simulink model "BSC_sfun"  (R2015b)
settings: Solver=FixedStepDiscrete  StartTime=0.0  StopTime=inf  FixedStep=bsck_stepSize  RelTol=1e-3
settings Model: TunableVars=bscv_LowFaultType,bscv_MediumFaultType,bscv_SevereFaultType  TunableVarsStorageClass=Auto,Auto,Auto  TunableVarsTypeQualifier=,,  Creator=nctzv8  LastModifiedBy=nctzv8
settings ConfigSet: Description=OpenECU configuration set for code generation under RTW-EC.
settings SolverCC: PositivePriorityOrder=on
settings DataIOCC: SaveFormat=Array  SignalLoggingSaveFormat=ModelDataLogs
settings OptimizationCC: DefaultParameterBehavior=Inlined  InlineInvariantSignals=on  ExpressionDepthLimit=2147483647  StateBitsets=on  DataBitsets=on  ZeroExternalMemoryAtStartup=off  ZeroInternalMemoryAtStartup=off  NoFixptDivByZeroProtection=on  EfficientFloat2IntCast=on  OptimizeModelRefInitCode=on  LifeSpan=1
settings DebuggingCC: SaveWithParameterizedLinksMsg=none  UnderspecifiedInitializationDetection=Classic  MergeDetectMultiDrivingBlocksExec=none  SignalResolutionControl=TryResolveAllWithWarning  MultiTaskDSMMsg=warning  MultiTaskCondExecSysMsg=none  SingleTaskRateTransMsg=error  CheckMatrixSingularityMsg=warning  VectorMatrixConversionMsg=warning  FcnCallInpInsideContextMsg=UseLocalSettings  SignalLabelMismatchMsg=warning  StateNameClashWarn=warning  StrictBusMsg=None
settings HardwareCC: ProdBitPerPointer=32  ProdLargestAtomicInteger=Long  ProdLargestAtomicFloat=Double  ProdEndianess=BigEndian  ProdWordSize=32  ProdHWDeviceType=Freescale->32-bit PowerPC  TargetIntDivRoundTo=Zero  TargetEndianess=BigEndian  TargetHWDeviceType=Freescale->32-bit PowerPC  ProdEqTarget=off
settings RTWCC: SystemTargetFile=openecu_ert.tlc  MakeCommand=make_rtw optimized_floating_point=1  TemplateMakefile=openecu_ert_r2015b_64.tmf  Description=OpenECU Platform Target (ERT, optimised floating-point code)  RetainRTWFile=on  IncludeHyperlinkInReport=on
settings CodeAppCC: ForceParamTrailComments=on  IgnoreCustomStorageClasses=off  SimulinkDataObjDesc=on  CustomSymbolStrType=$N$R$M  InsertBlockDesc=on  InternalIdentifier=Classic
settings STFCustomTargetCC: TargetLibSuffix=.a  GenerateSampleERTMain=on  ConcurrentExecutionCompliant=off  IncludeMdlTerminateFcn=off  GeneratePreprocessorConditionals=Use local settings  CombineOutputUpdateFcns=on  IncludeFileDelimiter=UseQuote  ERTCustomFileBanners=on  SupportContinuousTime=off  MATLABClassNameForMDSCustomization=Simulink.SoftwareTarget.ERTCustomization  CPPClassGenCompliant=off  GRTInterface=off  SystemTargetFile=openecu_ert.tlc
settings ERTTargetCC: GenerateSampleERTMain=on  ParMdlRefBuildCompliant=off  CompOptLevelCompliant=off  ConcurrentExecutionCompliant=off  IncludeMdlTerminateFcn=off  ERTFirstTimeCompliant=off  IncludeFileDelimiter=UseQuote  SupportNonInlinedSFcns=on  ModelStepFunctionPrototypeControlCompliant=off  CPPClassGenCompliant=off  UseToolchainInfoCompliant=off  ExtModeMexFile=noextcomm  InlinedParameterPlacement=NonHierarchical  ERTSrcFileBannerTemplate=oe_code_c_template.cgt  ERTHdrFileBannerTemplate=oe_code_h_template.cgt  ERTDataSrcFileTemplate=oe_data_c_template.cgt  ERTDataHdrFileTemplate=oe_data_h_template.cgt  ERTCustomFileTemplate=example_file_process.tlc  GlobalDataDefinition=InSeparateSourceFile  GlobalDataReference=InSeparateHeaderFile  EnableUserReplacementTypes=on

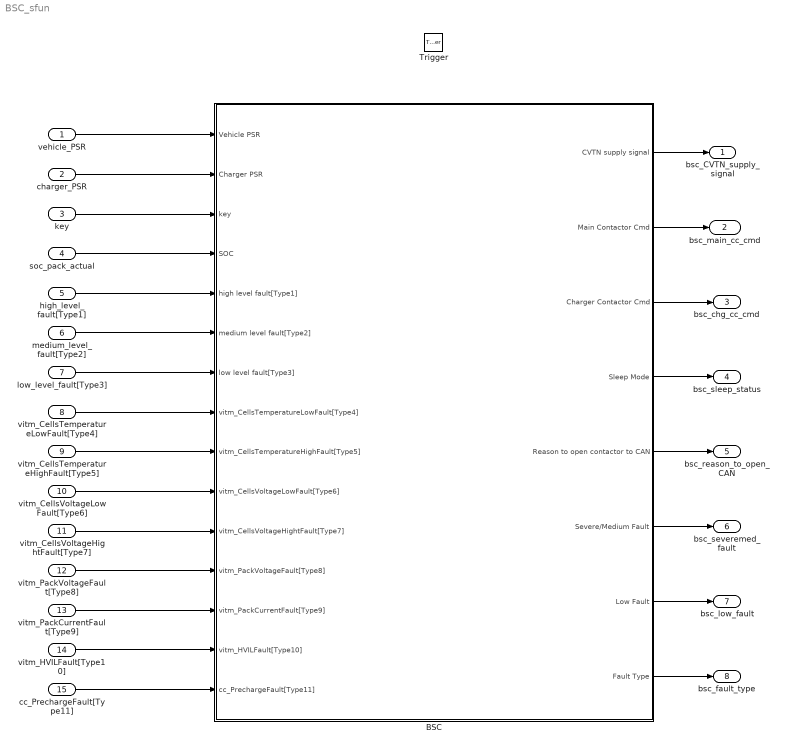
== system BSC_sfun ==
  vehicle_PSR : Inport  OutDataTypeStr=uint8  PortDimensions=1
  charger_PSR : Inport  Port=2  OutDataTypeStr=uint8  PortDimensions=1
  key : Inport  Port=3  OutDataTypeStr=uint8  PortDimensions=1
  soc_pack_actual : Inport  Port=4  OutDataTypeStr=double  PortDimensions=1
  high_level_fault[Type1] : Inport  Port=5  OutDataTypeStr=uint8  PortDimensions=1
  medium_level_fault[Type2] : Inport  Port=6  OutDataTypeStr=uint8  PortDimensions=1
  low_level_fault[Type3] : Inport  Port=7  OutDataTypeStr=uint8  PortDimensions=1
  vitm_CellsTemperatureLowFault[Type4] : Inport  Port=8  OutDataTypeStr=uint8  PortDimensions=1
  vitm_CellsTemperatureHighFault[Type5] : Inport  Port=9  OutDataTypeStr=uint8  PortDimensions=1
  vitm_CellsVoltageLowFault[Type6] : Inport  Port=10  OutDataTypeStr=uint8  PortDimensions=1
  vitm_CellsVoltageHightFault[Type7] : Inport  Port=11  OutDataTypeStr=uint8  PortDimensions=1
  vitm_PackVoltageFault[Type8] : Inport  Port=12  OutDataTypeStr=uint8  PortDimensions=1
  vitm_PackCurrentFault[Type9] : Inport  Port=13  OutDataTypeStr=uint8  PortDimensions=1
  vitm_HVILFault[Type10] : Inport  Port=14  OutDataTypeStr=uint8  PortDimensions=1
  cc_PrechargeFault[Type11] : Inport  Port=15  OutDataTypeStr=uint8  PortDimensions=1
  Trigger : TriggerPort  TriggerType=function-call  PortDimensions=1
  BSC : Subsystem
      mask help: Simulink:masks:GenSFuncDesc_MD
      mask Help: eval('feval(''rtwprivate'',''rtwhelpview'',''rtw_sfcn_block'')');
  bsc_CVTN_supply_signal : Outport  OutDataTypeStr=boolean  PortDimensions=1
  bsc_main_cc_cmd : Outport  Port=2  OutDataTypeStr=boolean  PortDimensions=1
  bsc_chg_cc_cmd : Outport  Port=3  OutDataTypeStr=boolean  PortDimensions=1
  bsc_sleep_status : Outport  Port=4  OutDataTypeStr=boolean  PortDimensions=1
  bsc_reason_to_open_CAN : Outport  Port=5  OutDataTypeStr=uint8  PortDimensions=1
  bsc_severemed_fault : Outport  Port=6  OutDataTypeStr=uint8  PortDimensions=1
  bsc_low_fault : Outport  Port=7  OutDataTypeStr=uint8  PortDimensions=1
  bsc_fault_type : Outport  Port=8  OutDataTypeStr=uint8  PortDimensions=1
  wires:
  vehicle_PSR/1 -> BSC/1(Vehicle PSR)
  charger_PSR/1 -> BSC/2(Charger PSR)
  key/1 -> BSC/3(key)
  soc_pack_actual/1 -> BSC/4(SOC)
  high_level_fault[Type1]/1 -> BSC/5(high level fault[Type1])
  medium_level_fault[Type2]/1 -> BSC/6(medium level fault[Type2])
  low_level_fault[Type3]/1 -> BSC/7(low level fault[Type3])
  vitm_CellsTemperatureLowFault[Type4]/1 -> BSC/8(vitm_CellsTemperatureLowFault[Type4])
  vitm_CellsTemperatureHighFault[Type5]/1 -> BSC/9(vitm_CellsTemperatureHighFault[Type5])
  vitm_CellsVoltageLowFault[Type6]/1 -> BSC/10(vitm_CellsVoltageLowFault[Type6])
  vitm_CellsVoltageHightFault[Type7]/1 -> BSC/11(vitm_CellsVoltageHightFault[Type7])
  vitm_PackVoltageFault[Type8]/1 -> BSC/12(vitm_PackVoltageFault[Type8])
  vitm_PackCurrentFault[Type9]/1 -> BSC/13(vitm_PackCurrentFault[Type9])
  cc_PrechargeFault[Type11]/1 -> BSC/15(cc_PrechargeFault[Type11])
  vitm_HVILFault[Type10]/1 -> BSC/14(vitm_HVILFault[Type10])
  BSC/1(CVTN supply signal) -> bsc_CVTN_supply_signal/1
  BSC/2(Main Contactor Cmd) -> bsc_main_cc_cmd/1
  BSC/3(Charger Contactor Cmd) -> bsc_chg_cc_cmd/1
  BSC/4(Sleep Mode) -> bsc_sleep_status/1
  BSC/5(Reason to open contactor to CAN) -> bsc_reason_to_open_CAN/1
  BSC/6(Severe/Medium Fault) -> bsc_severemed_fault/1
  BSC/7(Low Fault) -> bsc_low_fault/1
  BSC/8(Fault Type) -> bsc_fault_type/1

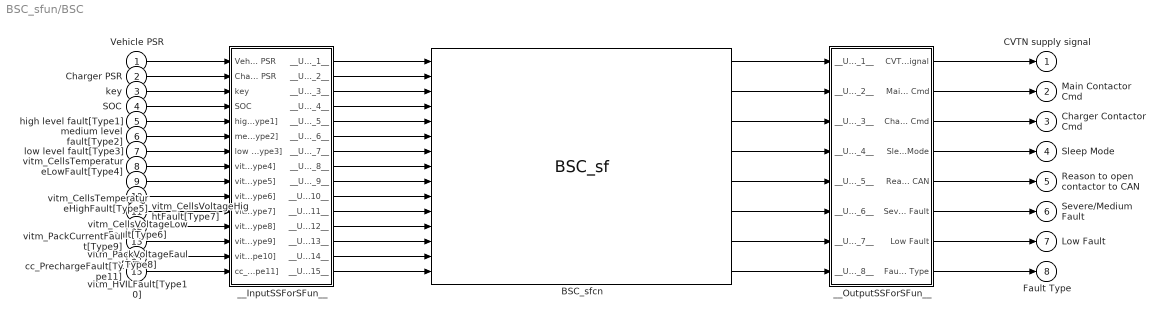
== system BSC_sfun/BSC ==
  Vehicle PSR : Inport  OutDataTypeStr=uint8  PortDimensions=1
  Charger PSR : Inport  Port=2  OutDataTypeStr=uint8  PortDimensions=1
  key : Inport  Port=3  OutDataTypeStr=uint8  PortDimensions=1
  SOC : Inport  Port=4  OutDataTypeStr=double  PortDimensions=1
  high level fault[Type1] : Inport  Port=5  OutDataTypeStr=uint8  PortDimensions=1
  medium level fault[Type2] : Inport  Port=6  OutDataTypeStr=uint8  PortDimensions=1
  low level fault[Type3] : Inport  Port=7  OutDataTypeStr=uint8  PortDimensions=1
  vitm_CellsTemperatureLowFault[Type4] : Inport  Port=8  OutDataTypeStr=uint8  PortDimensions=1
  vitm_CellsTemperatureHighFault[Type5] : Inport  Port=9  OutDataTypeStr=uint8  PortDimensions=1
  vitm_CellsVoltageLowFault[Type6] : Inport  Port=10  OutDataTypeStr=uint8  PortDimensions=1
  vitm_CellsVoltageHightFault[Type7] : Inport  Port=11  OutDataTypeStr=uint8  PortDimensions=1
  vitm_PackVoltageFault[Type8] : Inport  Port=12  OutDataTypeStr=uint8  PortDimensions=1
  vitm_PackCurrentFault[Type9] : Inport  Port=13  OutDataTypeStr=uint8  PortDimensions=1
  vitm_HVILFault[Type10] : Inport  Port=14  OutDataTypeStr=uint8  PortDimensions=1
  cc_PrechargeFault[Type11] : Inport  Port=15  OutDataTypeStr=uint8  PortDimensions=1
  BSC_sfcn : S-Function  FunctionName=BSC_sf  SFunctionModules=""  SFunctionDeploymentMode=off  EnableBusSupport=off  mask{rtw_sf_name=BSC_sf, showVar=off}
      mask prompts: rtw_sf_name "Simulink:masks:GenSFuncName_MP"; showVar "Simulink:masks:GenSFuncShowModuleList_MP"
      mask help: Simulink:masks:GenSFuncDesc_MD
      mask init:
      | displist = '';
      | if ~strcmp(get_param(gcb, 'FunctionName'), rtw_sf_name);
      |   set_param(gcb, 'FunctionName', rtw_sf_name);
      | end
      | % Check if we are generating code
      | rtw_mode = false;
      | if strcmpi(get_param(bdroot(gcb),'SimulationStatus'),'Initializing')
      | 	rtw_mode = strcmpi(get_param(bdroot(gcb),'BuildingRTWCode'),'on') && ...
      | 		~strcmpi(get_param(bdroot(gcb),'TargetStyle'),'SimulationTarget');
      | end
      | if showVar || rtw_mode
      | 	if exist('rtwsfunc') == 2 | exist('rtwsfunc') == 6
      | 		tmplist = rtwsfunc(rtw_sf_name,gcb);
      | 		tmplist = DAStudio.message('Simulink:masks:GenSFuncListOfModules_IC', tmplist);
      | 	elseif showVar
      | 		tmplist1 = DAStudio.message('Simulink:masks:GenSFuncListOfModules_IC', '');
      |         tmplist2 = DAStudio.message('Simulink:masks:GenSFuncNotLicensed_IC');
      |         tmplist = [tmplist1 tmplist2];
      |  	end
      | end
      | if showVar
      |   displist = tmplist;
      | end
      settings: CopyFcn=|
      | if ~strcmp(get_param(gcb,'Linkstatus'),'none') && ...
      | ~strcmp(get_param(gcb,'Linkstatus'),'implicit')
      |   set_param(gcb,'LinkStatus','none');
      | end
      mask Help: eval('feval(''rtwprivate'',''rtwhelpview'',''rtw_sfcn_block'')');
      mask Display:
      | port_label('input',1,'Vehicle PSR');
      | port_label('input',2,'Charger PSR');
      | port_label('input',3,'key');
      | port_label('input',4,'SOC');
      | port_label('input',5,'high level fault[Type1]');
      | port_label('input',6,'medium level fault[Type2]');
      | port_label('input',7,'low level fault[Type3]');
      | port_label('input',8,'vitm_CellsTemperatureLowFault[Type4]');
      | port_label('input',9,'vitm_CellsTemperatureHighFault[Type5]');
      | port_label('input',10,'vitm_CellsVoltageLowFault[Type6]');
      | port_label('input',11,'vitm_CellsVoltageHightFault[Type7]');
      | port_label('input',12,'vitm_PackVoltageFault[Type8]');
      | port_label('input',13,'vitm_PackCurrentFault[Type9]');
      | port_label('input',14,'vitm_HVILFault[Type10]');
      | port_label('input',15,'cc_PrechargeFault[Type11]');
      | port_label('output',1,'CVTN supply signal');
      | port_label('output',2,'Main Contactor Cmd');
      | port_label('output',3,'Charger Contactor Cmd');
      | port_label('output',4,'Sleep Mode');
      | port_label('output',5,'Reason to open contactor to CAN');
      | port_label('output',6,'Severe/Medium Fault');
      | port_label('output',7,'Low Fault');
      | port_label('output',8,'Fault Type');
  __InputSSForSFun__ : Subsystem
  __OutputSSForSFun__ : Subsystem
  CVTN supply signal : Outport  OutDataTypeStr=boolean  PortDimensions=1
  Main Contactor Cmd : Outport  Port=2  OutDataTypeStr=boolean  PortDimensions=1
  Charger Contactor Cmd : Outport  Port=3  OutDataTypeStr=boolean  PortDimensions=1
  Sleep Mode : Outport  Port=4  OutDataTypeStr=boolean  PortDimensions=1
  Reason to open contactor to CAN : Outport  Port=5  OutDataTypeStr=uint8  PortDimensions=1
  Severe/Medium Fault : Outport  Port=6  OutDataTypeStr=uint8  PortDimensions=1
  Low Fault : Outport  Port=7  OutDataTypeStr=uint8  PortDimensions=1
  Fault Type : Outport  Port=8  OutDataTypeStr=uint8  PortDimensions=1
  wires:
  Vehicle PSR/1 -> __InputSSForSFun__/1(Vehicle PSR)
  Charger PSR/1 -> __InputSSForSFun__/2(Charger PSR)
  key/1 -> __InputSSForSFun__/3(key)
  SOC/1 -> __InputSSForSFun__/4(SOC)
  high level fault[Type1]/1 -> __InputSSForSFun__/5(high level fault[Type1])
  medium level fault[Type2]/1 -> __InputSSForSFun__/6(medium level fault[Type2])
  low level fault[Type3]/1 -> __InputSSForSFun__/7(low level fault[Type3])
  vitm_CellsTemperatureLowFault[Type4]/1 -> __InputSSForSFun__/8(vitm_CellsTemperatureLowFault[Type4])
  vitm_CellsTemperatureHighFault[Type5]/1 -> __InputSSForSFun__/9(vitm_CellsTemperatureHighFault[Type5])
  vitm_CellsVoltageLowFault[Type6]/1 -> __InputSSForSFun__/10(vitm_CellsVoltageLowFault[Type6])
  vitm_CellsVoltageHightFault[Type7]/1 -> __InputSSForSFun__/11(vitm_CellsVoltageHightFault[Type7])
  vitm_PackVoltageFault[Type8]/1 -> __InputSSForSFun__/12(vitm_PackVoltageFault[Type8])
  vitm_PackCurrentFault[Type9]/1 -> __InputSSForSFun__/13(vitm_PackCurrentFault[Type9])
  vitm_HVILFault[Type10]/1 -> __InputSSForSFun__/14(vitm_HVILFault[Type10])
  cc_PrechargeFault[Type11]/1 -> __InputSSForSFun__/15(cc_PrechargeFault[Type11])
  __InputSSForSFun__/1(__UniqueOutportName__1__) -> BSC_sfcn/1
  __InputSSForSFun__/2(__UniqueOutportName__2__) -> BSC_sfcn/2
  __InputSSForSFun__/3(__UniqueOutportName__3__) -> BSC_sfcn/3
  __InputSSForSFun__/4(__UniqueOutportName__4__) -> BSC_sfcn/4
  __InputSSForSFun__/5(__UniqueOutportName__5__) -> BSC_sfcn/5
  __InputSSForSFun__/6(__UniqueOutportName__6__) -> BSC_sfcn/6
  __InputSSForSFun__/7(__UniqueOutportName__7__) -> BSC_sfcn/7
  __InputSSForSFun__/8(__UniqueOutportName__8__) -> BSC_sfcn/8
  __InputSSForSFun__/9(__UniqueOutportName__9__) -> BSC_sfcn/9
  __InputSSForSFun__/10(__UniqueOutportName__10__) -> BSC_sfcn/10
  __InputSSForSFun__/11(__UniqueOutportName__11__) -> BSC_sfcn/11
  __InputSSForSFun__/12(__UniqueOutportName__12__) -> BSC_sfcn/12
  __InputSSForSFun__/13(__UniqueOutportName__13__) -> BSC_sfcn/13
  __InputSSForSFun__/14(__UniqueOutportName__14__) -> BSC_sfcn/14
  __InputSSForSFun__/15(__UniqueOutportName__15__) -> BSC_sfcn/15
  BSC_sfcn/1 -> __OutputSSForSFun__/1(__UniqueInportName__1__)
  BSC_sfcn/2 -> __OutputSSForSFun__/2(__UniqueInportName__2__)
  BSC_sfcn/3 -> __OutputSSForSFun__/3(__UniqueInportName__3__)
  BSC_sfcn/4 -> __OutputSSForSFun__/4(__UniqueInportName__4__)
  BSC_sfcn/5 -> __OutputSSForSFun__/5(__UniqueInportName__5__)
  BSC_sfcn/6 -> __OutputSSForSFun__/6(__UniqueInportName__6__)
  BSC_sfcn/7 -> __OutputSSForSFun__/7(__UniqueInportName__7__)
  BSC_sfcn/8 -> __OutputSSForSFun__/8(__UniqueInportName__8__)
  __OutputSSForSFun__/1(CVTN supply signal) -> CVTN supply signal/1
  __OutputSSForSFun__/2(Main Contactor Cmd) -> Main Contactor Cmd/1
  __OutputSSForSFun__/3(Charger Contactor Cmd) -> Charger Contactor Cmd/1
  __OutputSSForSFun__/4(Sleep Mode) -> Sleep Mode/1
  __OutputSSForSFun__/5(Reason to open contactor to CAN) -> Reason to open contactor to CAN/1
  __OutputSSForSFun__/6(Severe/Medium Fault) -> Severe/Medium Fault/1
  __OutputSSForSFun__/7(Low Fault) -> Low Fault/1
  __OutputSSForSFun__/8(Fault Type) -> Fault Type/1

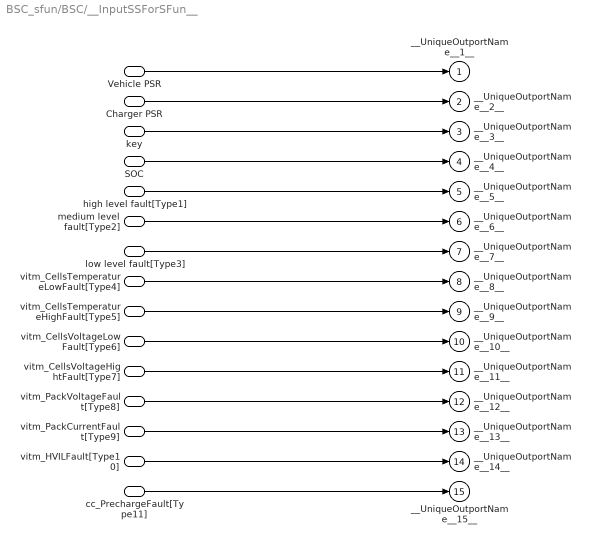
== system BSC_sfun/BSC/__InputSSForSFun__ ==
  Vehicle PSR : Inport  OutDataTypeStr=uint8  PortDimensions=1
  Charger PSR : Inport  Port=2  OutDataTypeStr=uint8  PortDimensions=1
  key : Inport  Port=3  OutDataTypeStr=uint8  PortDimensions=1
  SOC : Inport  Port=4  OutDataTypeStr=double  PortDimensions=1
  high level fault[Type1] : Inport  Port=5  OutDataTypeStr=uint8  PortDimensions=1
  medium level fault[Type2] : Inport  Port=6  OutDataTypeStr=uint8  PortDimensions=1
  low level fault[Type3] : Inport  Port=7  OutDataTypeStr=uint8  PortDimensions=1
  vitm_CellsTemperatureLowFault[Type4] : Inport  Port=8  OutDataTypeStr=uint8  PortDimensions=1
  vitm_CellsTemperatureHighFault[Type5] : Inport  Port=9  OutDataTypeStr=uint8  PortDimensions=1
  vitm_CellsVoltageLowFault[Type6] : Inport  Port=10  OutDataTypeStr=uint8  PortDimensions=1
  vitm_CellsVoltageHightFault[Type7] : Inport  Port=11  OutDataTypeStr=uint8  PortDimensions=1
  vitm_PackVoltageFault[Type8] : Inport  Port=12  OutDataTypeStr=uint8  PortDimensions=1
  vitm_PackCurrentFault[Type9] : Inport  Port=13  OutDataTypeStr=uint8  PortDimensions=1
  vitm_HVILFault[Type10] : Inport  Port=14  OutDataTypeStr=uint8  PortDimensions=1
  cc_PrechargeFault[Type11] : Inport  Port=15  OutDataTypeStr=uint8  PortDimensions=1
  __UniqueOutportName__1__ : Outport
  __UniqueOutportName__2__ : Outport  Port=2
  __UniqueOutportName__3__ : Outport  Port=3
  __UniqueOutportName__4__ : Outport  Port=4
  __UniqueOutportName__5__ : Outport  Port=5
  __UniqueOutportName__6__ : Outport  Port=6
  __UniqueOutportName__7__ : Outport  Port=7
  __UniqueOutportName__8__ : Outport  Port=8
  __UniqueOutportName__9__ : Outport  Port=9
  __UniqueOutportName__10__ : Outport  Port=10
  __UniqueOutportName__11__ : Outport  Port=11
  __UniqueOutportName__12__ : Outport  Port=12
  __UniqueOutportName__13__ : Outport  Port=13
  __UniqueOutportName__14__ : Outport  Port=14
  __UniqueOutportName__15__ : Outport  Port=15
  wires:
  Vehicle PSR/1 -> __UniqueOutportName__1__/1
  Charger PSR/1 -> __UniqueOutportName__2__/1
  key/1 -> __UniqueOutportName__3__/1
  SOC/1 -> __UniqueOutportName__4__/1
  high level fault[Type1]/1 -> __UniqueOutportName__5__/1
  medium level fault[Type2]/1 -> __UniqueOutportName__6__/1
  low level fault[Type3]/1 -> __UniqueOutportName__7__/1
  vitm_CellsTemperatureLowFault[Type4]/1 -> __UniqueOutportName__8__/1
  vitm_CellsTemperatureHighFault[Type5]/1 -> __UniqueOutportName__9__/1
  vitm_CellsVoltageLowFault[Type6]/1 -> __UniqueOutportName__10__/1
  vitm_CellsVoltageHightFault[Type7]/1 -> __UniqueOutportName__11__/1
  vitm_PackVoltageFault[Type8]/1 -> __UniqueOutportName__12__/1
  vitm_PackCurrentFault[Type9]/1 -> __UniqueOutportName__13__/1
  vitm_HVILFault[Type10]/1 -> __UniqueOutportName__14__/1
  cc_PrechargeFault[Type11]/1 -> __UniqueOutportName__15__/1

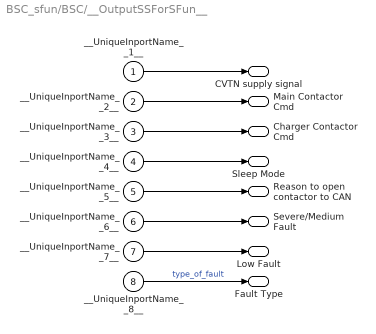
== system BSC_sfun/BSC/__OutputSSForSFun__ ==
  __UniqueInportName__1__ : Inport
  __UniqueInportName__2__ : Inport  Port=2
  __UniqueInportName__3__ : Inport  Port=3
  __UniqueInportName__4__ : Inport  Port=4
  __UniqueInportName__5__ : Inport  Port=5
  __UniqueInportName__6__ : Inport  Port=6
  __UniqueInportName__7__ : Inport  Port=7
  __UniqueInportName__8__ : Inport  Port=8
  CVTN supply signal : Outport  OutDataTypeStr=boolean  PortDimensions=1
  Main Contactor Cmd : Outport  Port=2  OutDataTypeStr=boolean  PortDimensions=1
  Charger Contactor Cmd : Outport  Port=3  OutDataTypeStr=boolean  PortDimensions=1
  Sleep Mode : Outport  Port=4  OutDataTypeStr=boolean  PortDimensions=1
  Reason to open contactor to CAN : Outport  Port=5  OutDataTypeStr=uint8  PortDimensions=1
  Severe/Medium Fault : Outport  Port=6  OutDataTypeStr=uint8  PortDimensions=1
  Low Fault : Outport  Port=7  OutDataTypeStr=uint8  PortDimensions=1
  Fault Type : Outport  Port=8  OutDataTypeStr=uint8  PortDimensions=1
  wires:
  __UniqueInportName__1__/1 -> CVTN supply signal/1
  __UniqueInportName__2__/1 -> Main Contactor Cmd/1
  __UniqueInportName__3__/1 -> Charger Contactor Cmd/1
  __UniqueInportName__4__/1 -> Sleep Mode/1
  __UniqueInportName__5__/1 -> Reason to open contactor to CAN/1
  __UniqueInportName__6__/1 -> Severe/Medium Fault/1
  __UniqueInportName__7__/1 -> Low Fault/1
  __UniqueInportName__8__/1 -> Fault Type/1  "type_of_fault"
